simulink model "control_test"  (R2018b)
settings: Solver=ode45  StartTime=0.0  StopTime=900  RelTol=1e-3
values from neighbouring files (symbols this model uses):
  P = struct    [controller_test_main.m]
  q0 = q0/norm(q0)    [controller_test_main.m]
  qd = qd/norm(qd)    [controller_test_main.m]
  w0 = [0; 0; 0]    [controller_test_main.m]
undefined symbols (not defined in the file or in its folder): satelliteDynamics_lib
libraries: control_gen x1, vrlib x1, aerolibutil x1
settings Model: Creator=colem  LastModifiedBy=colem

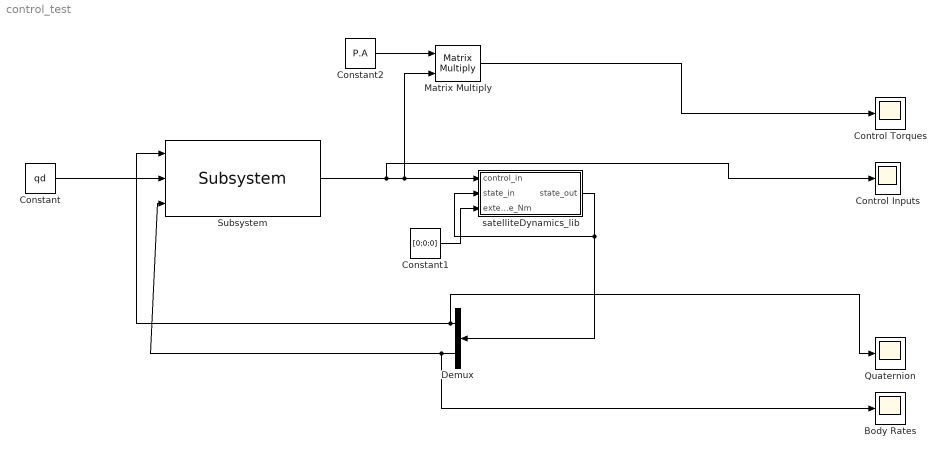
== system control_test ==
  Body Rates : Scope
  Constant : Constant  Value=qd
  Constant1 : Constant  Value=[0;0;0]
  Constant2 : Constant  Value=P.A
  Control Inputs : Scope
  Control Torques : Scope
  Demux : Demux  Outputs=[4 3]
  Matrix Multiply : Product  Multiplication=Matrix(*)
  Quaternion : Scope
  Subsystem : control_gen/Subsystem  SystemSampleTime=-1
  satelliteDynamics_lib : Subsystem  AncestorBlock=satelliteDynamics_lib/satelliteDynamics_lib
  wires:
  Subsystem/1 -> Matrix Multiply/2, satelliteDynamics_lib/1(control_in), Control Inputs/1
  satelliteDynamics_lib/1(state_out) -> satelliteDynamics_lib/2(state_in), Demux/1
  Constant/1 -> Subsystem/2
  Constant1/1 -> satelliteDynamics_lib/3(external_torque_Nm)
  Demux/1 -> Quaternion/1, Subsystem/1
  Demux/2 -> Body Rates/1, Subsystem/3
  Constant2/1 -> Matrix Multiply/1
  Matrix Multiply/1 -> Control Torques/1

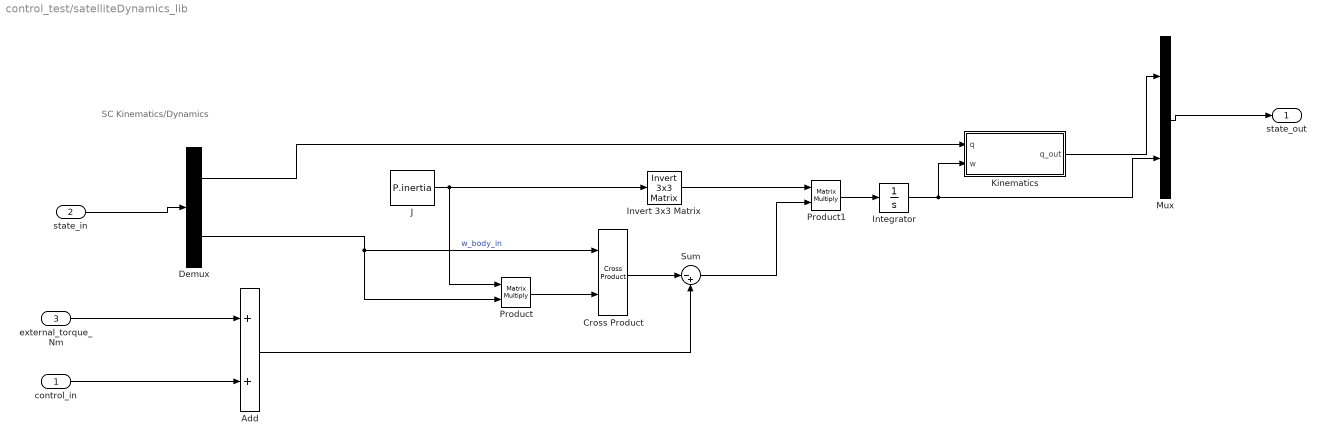
== system control_test/satelliteDynamics_lib ==
  note: SC Kinematics/Dynamics
  control_in : Inport
  state_in : Inport  Port=2
  external_torque_Nm : Inport  Port=3
  Add : Sum
  Cross Product : vrlib/Utilities/Cross Product
      settings: SourceProductBaseCode=VR
  Demux : Demux  Outputs=[4 3]
  Integrator : Integrator  InitialCondition=w0
  Invert 3x3 Matrix : aerolibutil/Invert  3x3 Matrix
  J : Constant  Value=P.inertia
  Kinematics : Subsystem
  Mux : Mux  Inputs=[4 3]
  Product : Product  Multiplication=Matrix(*)
  Product1 : Product  Multiplication=Matrix(*)
  Sum : Sum  Inputs=|-+
  state_out : Outport
  wires:
  J/1 -> Product/1, Invert 3x3 Matrix/1
  Product/1 -> Cross Product/2
  Cross Product/1 -> Sum/1
  Sum/1 -> Product1/2
  Invert 3x3 Matrix/1 -> Product1/1
  Product1/1 -> Integrator/1
  Integrator/1 -> Mux/2, Kinematics/2(w)
  Kinematics/1(q_out) -> Mux/1
  Demux/2 -> Cross Product/1, Product/2  "w_body_in"
  Demux/1 -> Kinematics/1(q)
  Mux/1 -> state_out/1
  state_in/1 -> Demux/1
  external_torque_Nm/1 -> Add/1
  control_in/1 -> Add/2
  Add/1 -> Sum/2

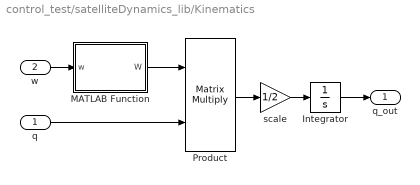
== system control_test/satelliteDynamics_lib/Kinematics ==
  q : Inport
  w : Inport  Port=2
  Integrator : Integrator  InitialCondition=q0
  MATLAB Function : MATLAB Function  TreatAsAtomicUnit=on
  Product : Product  Multiplication=Matrix(*)
  scale : Gain  Gain=1/2
  q_out : Outport
  wires:
  w/1 -> MATLAB Function/1(w)
  MATLAB Function/1(W) -> Product/1
  q/1 -> Product/2
  Product/1 -> scale/1
  scale/1 -> Integrator/1
  Integrator/1 -> q_out/1

== matlab function control_test/satelliteDynamics_lib/Kinematics/MATLAB Function ==
  data: w input; W output
function W = fcn(w)
%#codegen

W = [0, -w(1),-w(2),-w(3); w(1), 0,w(3), -w(2); w(2), -w(3), 0, w(1); w(3), w(2), -w(1), 0 ];

end
